simulink model "Smart_Grid_2"  (R2024b)
settings: Solver=FixedStepAuto  StartTime=0.0  StopTime=0.5  FixedStep=1e-5  RelTol=1e-3
undefined symbols (not defined in the file): Ion, Lithium
libraries: spsSeriesRLCBranchLib x76, spsRMSLib x65, spsIGBTDiodeLib x41, eeGeneralControl x36, slpidlib x34, spsThreePhaseVIMeasurementLib x32, spsVoltageMeasurementLib x18, simulink x16, spsCurrentMeasurementLib x15, spsThreePhaseBreakerLib x12, spsAlphaBetaZerotodq0Lib x12, spsPower3phPhasorLib x10
(part 1 of 8)
settings Model: Creator=siva kumar  LastModifiedBy=siva kumar
settings RTWCC: GPUComputeCapability=3.5

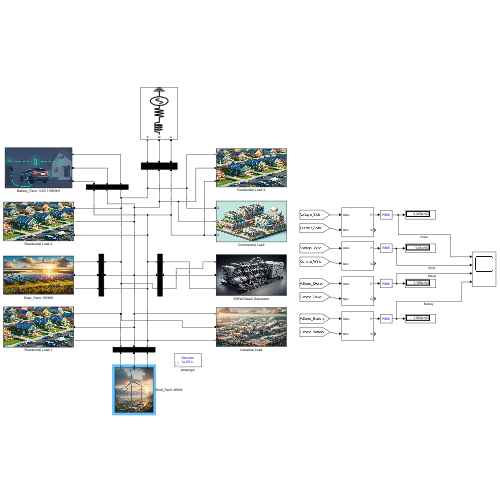
[thumbnail: Simulink's stored preview of the top-level diagram]
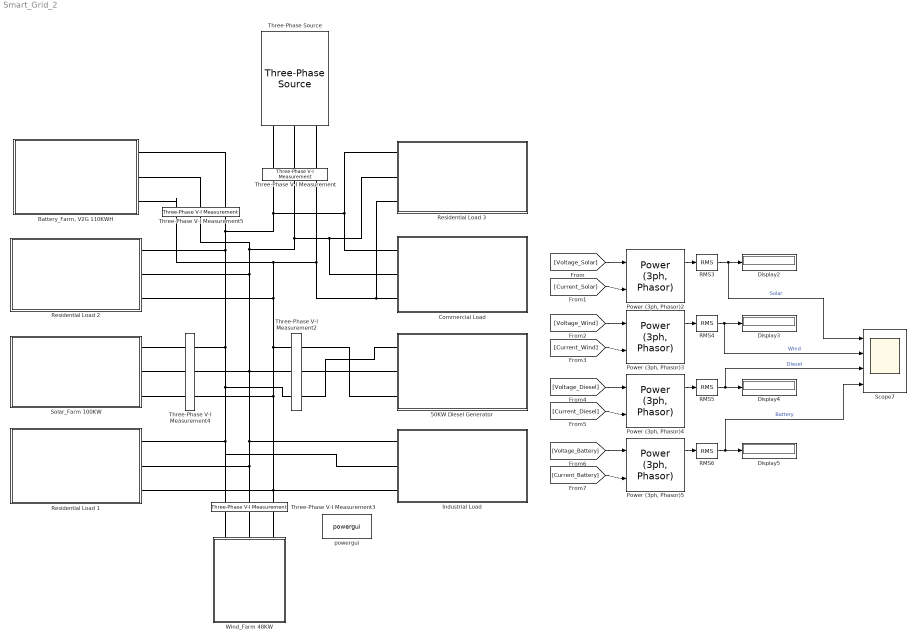
== system Smart_Grid_2 ==
  50KW Diesel Generator : Subsystem
      mask Display: image('Diesel_Image.jpg');
  "Battery_Farm, V2G 110KWH" : Subsystem
      mask Display: image('v2g.png');
  Commercial Load : Subsystem
      mask Display: image('Commercial_Image.jpg');
  Display{2..5} (4 alike) : Display
  Industrial Load : Subsystem
      mask Display: image('Industrial_Image.jpg');
  Power (3ph, Phasor){2..5} (4 alike) : spsPower3phPhasorLib/Power (3ph, Phasor)
      settings: LibrarySourceBlock=|
      | sps_lib/Sensors and Measurements/Power
      | (3ph, Phasor)
  RMS{3..6} (4 alike) : spsRMSLib/RMS  TrueRMS=on  Freq=50  RMSInit=0  Ts=0
  Residential Load 1 : Subsystem
      mask Display: image('Residential_Image.jpg');
  Residential Load 2 : Subsystem
      mask Display: image('Residential_Image.jpg');
  Residential Load 3 : Subsystem
      mask Display: image('Residential_Image.jpg');
  Scope7 : Scope  NumInputPorts=4
  Solar_Farm 100KW : Subsystem
      mask Display: image('Solar_Image.jpg');
  Three-Phase V-I Measurement : spsThreePhaseVIMeasurementLib/Three-Phase V-I Measurement  VoltageMeasurement=phase-to-ground  SetLabelV=on  LabelV=Grid_Voltage  Vpu=off  VpuLL=off  CurrentMeasurement=yes  SetLabelI=on  LabelI=Grid_Current  Ipu=off  Pbase=100e6  Vbase=500e3  OutputType=Complex  PhasorSimulation=off  PSBequivalent=0
  Three-Phase V-I Measurement2 : spsThreePhaseVIMeasurementLib/Three-Phase V-I Measurement  VoltageMeasurement=phase-to-ground  SetLabelV=on  LabelV=Voltage_Diesel  Vpu=off  VpuLL=off  CurrentMeasurement=yes  SetLabelI=on  LabelI=Current_Diesel  Ipu=off  Pbase=100e6  Vbase=500e3  OutputType=Complex  PhasorSimulation=off  PSBequivalent=0
  Three-Phase V-I Measurement3 : spsThreePhaseVIMeasurementLib/Three-Phase V-I Measurement  VoltageMeasurement=phase-to-ground  SetLabelV=on  LabelV=Voltage_Wind  Vpu=off  VpuLL=off  CurrentMeasurement=yes  SetLabelI=on  LabelI=Current_Wind  Ipu=off  Pbase=100e6  Vbase=500e3  OutputType=Complex  PhasorSimulation=off  PSBequivalent=0
  Three-Phase V-I Measurement4 : spsThreePhaseVIMeasurementLib/Three-Phase V-I Measurement  VoltageMeasurement=phase-to-ground  SetLabelV=on  LabelV=Voltage_Solar  Vpu=off  VpuLL=off  CurrentMeasurement=yes  SetLabelI=on  LabelI=Current_Solar  Ipu=off  Pbase=100e6  Vbase=500e3  OutputType=Complex  PhasorSimulation=off  PSBequivalent=0
  Three-Phase V-I Measurement5 : spsThreePhaseVIMeasurementLib/Three-Phase V-I Measurement  VoltageMeasurement=phase-to-ground  SetLabelV=on  LabelV=Voltage_Battery  Vpu=off  VpuLL=off  CurrentMeasurement=yes  SetLabelI=on  LabelI=Current_Battery  Ipu=off  Pbase=100e6  Vbase=500e3  OutputType=Complex  PhasorSimulation=off  PSBequivalent=0
  Three-Phase Source : spsThreePhaseSourceLib/Three-Phase Source  InternalConnection=Yg  VoltagePhases=off  Voltage=25e3  PhaseAngle=0  Voltage_phases=[25e3 25e3 25e3]/sqrt(3)  PhaseAngles_phases=[0 -120 +120]  Frequency=50  NonIdealSource=on  SpecifyImpedance=off  Resistance=0.8929  Inductance=16.58e-3  ShortCircuitLevel=100e6  BaseVoltage=25e3  XRratio=7  BusType=swing  Pref=10e3  Qref=0  Prefabc=[10e3, 10e3, 10e3]  Qrefabc=[0, 0, 0]  Qmin=-inf  Qmax=inf
  Wind_Farm 48KW : Subsystem
      mask Display: image('Wind_Image.jpg');
  powergui : sps_lib/powergui  Priority=1  SimulationMode=Discrete  SampleTime=1e-5  frequency=60  Iterations=50  frequencyindice=0  Pbase=100e6  ErrMax=1e-4  UnitsV=kV  UnitsW=MW  buscounter=0  FunctionMessages=off  echomessages=off  EnableUseOfTLC=off  CurrentSourceSwitches=off  DisableSnubberDevices=off  DisableRonSwitches=off  DisableVfSwitches=off  DisplayEquations=off  AutomaticDiscreteSolvers=off  SolverType=Tustin/Backward Euler (TBE)  Interpol=off  ExternalGateDelay=off  methode=off  Ts=100  x0status=blocks  SPID=on  SwTol=0  HookPort=off  NonlinearTolerance=1e-4  nMaxIteration=100  ContinueOnMaxIteration=off  RestoreLinks=warning  ResistiveCurrentMeasurement=off  Frange=[0:2:500]  Ylog=off  Xlog=on  ShowGrid=off  save=off  variable=ZData  structure=0  ZoomFFT=off  StartTime=0.0  cycles=1  DisplayStyle=1  fundamental=60  FreqAxis=off  MaxFrequency=1000  frequencyindicesteady=1  RmsSteady=1  display=off
  wires:
  RMS3/1 -> Scope7/1, Display2/1  "Solar"
  "Power (3ph, Phasor)2"/1 -> RMS3/1
  [Voltage_Solar] -> "Power (3ph, Phasor)2"/1
  [Current_Solar] -> "Power (3ph, Phasor)2"/2
  [Current_Wind] -> "Power (3ph, Phasor)3"/2
  [Voltage_Wind] -> "Power (3ph, Phasor)3"/1
  "Power (3ph, Phasor)3"/1 -> RMS4/1
  RMS4/1 -> Scope7/2, Display3/1  "Wind"
  RMS5/1 -> Scope7/3, Display4/1  "Diesel"
  "Power (3ph, Phasor)4"/1 -> RMS5/1
  [Voltage_Diesel] -> "Power (3ph, Phasor)4"/1
  [Current_Diesel] -> "Power (3ph, Phasor)4"/2
  [Current_Battery] -> "Power (3ph, Phasor)5"/2
  [Voltage_Battery] -> "Power (3ph, Phasor)5"/1
  "Power (3ph, Phasor)5"/1 -> RMS6/1
  RMS6/1 -> Scope7/4, Display5/1  "Battery"
  connections:
  Three-Phase V-I Measurement3/RConn1 -- Residential Load 2/LConn1 -- Residential Load 3/LConn1 -- Commercial Load/LConn1 -- Three-Phase V-I Measurement/RConn1 -- Three-Phase V-I Measurement5/RConn1 -- Three-Phase V-I Measurement4/RConn1 -- Three-Phase V-I Measurement2/RConn1 -- Industrial Load/LConn2 -- Residential Load 1/LConn1
  Three-Phase V-I Measurement2/RConn3 -- Residential Load 2/LConn3 -- Three-Phase V-I Measurement5/RConn3 -- Residential Load 3/LConn3 -- Commercial Load/LConn3 -- Three-Phase V-I Measurement/RConn3 -- Industrial Load/LConn3 -- Three-Phase V-I Measurement3/RConn3 -- Residential Load 1/LConn3 -- Three-Phase V-I Measurement4/RConn3
  Three-Phase V-I Measurement2/RConn2 -- Residential Load 2/LConn2 -- Three-Phase V-I Measurement5/RConn2 -- Residential Load 3/LConn2 -- Commercial Load/LConn2 -- Three-Phase V-I Measurement/RConn2 -- Three-Phase V-I Measurement3/RConn2 -- Residential Load 1/LConn2 -- Industrial Load/LConn1 -- Three-Phase V-I Measurement4/RConn2
  Three-Phase Source/RConn1 -- Three-Phase V-I Measurement/LConn1
  Three-Phase Source/RConn2 -- Three-Phase V-I Measurement/LConn2
  Three-Phase Source/RConn3 -- Three-Phase V-I Measurement/LConn3
  Wind_Farm 48KW/RConn2 -- Three-Phase V-I Measurement3/LConn2
  Wind_Farm 48KW/RConn1 -- Three-Phase V-I Measurement3/LConn1
  Solar_Farm 100KW/RConn1 -- Three-Phase V-I Measurement4/LConn1
  Solar_Farm 100KW/RConn2 -- Three-Phase V-I Measurement4/LConn2
  Solar_Farm 100KW/RConn3 -- Three-Phase V-I Measurement4/LConn3
  Three-Phase V-I Measurement5/LConn1 -- "Battery_Farm, V2G 110KWH"/RConn1
  Three-Phase V-I Measurement5/LConn2 -- "Battery_Farm, V2G 110KWH"/RConn2
  Three-Phase V-I Measurement5/LConn3 -- "Battery_Farm, V2G 110KWH"/RConn3
  Three-Phase V-I Measurement3/LConn3 -- Wind_Farm 48KW/RConn3
  Three-Phase V-I Measurement2/LConn1 -- 50KW Diesel Generator/RConn1
  Three-Phase V-I Measurement2/LConn2 -- 50KW Diesel Generator/RConn2
  Three-Phase V-I Measurement2/LConn3 -- 50KW Diesel Generator/RConn3

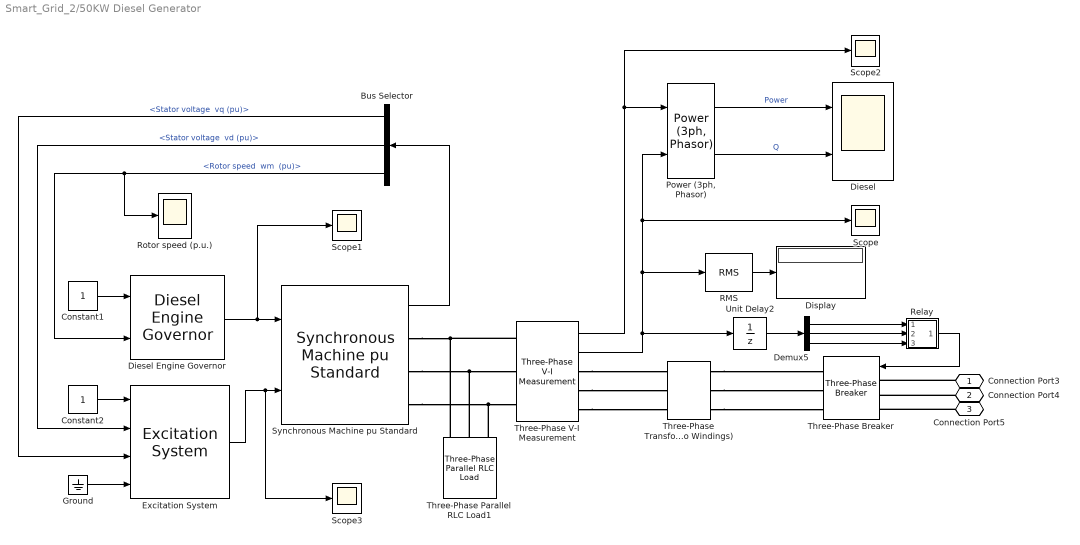
== system Smart_Grid_2/50KW Diesel Generator ==
  Bus Selector : BusSelector  OutputSignals="dq0 components.Stator voltage  vq (pu),dq0 components.Stator voltage  vd (pu),Mechanical.Rotor speed  wm  (pu)"
  Constant1 : Constant
  Constant2 : Constant
  Demux5 : Demux  Outputs=3
  Diesel : Scope  NumInputPorts=2
  Diesel Engine Governor : spsDieselMotorModel/Diesel Engine Governor  K=65  Tr=[0.01 0.02 0.2]  Ta=[0.25 0.009 0.0384]  Tlim=[0.1 1.1]  Td=0.020  Pm0=0.007343
  Display : Display
  Excitation System : spsExcitationSystemLib/Excitation System  tr=20e-3  reg=[ 300, 0.001 ]  exc=[ 1, 0 ]  tgr=[ 0, 0 ]  damp=[ 0.001, 0.1 ]  sat=[ 0, 0 ]  lim=[ -11.5, 11.5, 0 ]  v0=[1 1.0072]
      settings: LibrarySourceBlock=sps_lib/Electrical Machines/Synchronous Machine Control/Excitation System
  Ground : Ground
  "Power (3ph, Phasor)" : spsPower3phPhasorLib/Power (3ph, Phasor)
      settings: LibrarySourceBlock=|
      | sps_lib/Sensors and Measurements/Power
      | (3ph, Phasor)
  RMS : spsRMSLib/RMS  TrueRMS=on  Freq=50  RMSInit=0  Ts=0.001
  Relay : Subsystem
  Rotor speed (p.u.) : Scope
  Scope{,1..3} (4 alike) : Scope
  Synchronous Machine pu Standard : spsSynchronousMachinepuStandardLib/Synchronous Machine pu Standard  PresetModel=No  MechanicalLoad=Mechanical power Pm  ShowDetailedParameters=on  RotorType=Salient-pole  Units=per unit standard parameters  MeasurementBus=off  NominalParameters="[ 150e3  25e3   50]"  Reactances1=[ 1.81, 0.3, 0.23, 1.76, 0.65, 0.25, 0.15 ]  Reactances2="[ 1.305, 0.296, 0.252, 0.474,  0.243,  0.18 ]"  dAxisTimeConstants=Open-circuit  qAxisTimeConstants=Short-circuit  TimeConstants1="[ 4.4849  0.0681  0.1  ]"  TimeConstants2=[ 8.0, 0.03, 1.0, 0.07 ]  TimeConstants3="[  4.49  0.0681  0.0513  ]"  TimeConstants4=[ 8.0, 0.03, 0.3371, 0.0295 ]  TimeConstants5=[ 1.01, 0.053, 0.1 ]  TimeConstants6=[ 1.3201, 0.023, 1.0, 0.07 ]  TimeConstants7=[0.012 0.003 0.003]  TimeConstants8=[ 1.3201, 0.0231, 0.3371, 0.0295 ]  StatorResistance=0.003  Mechanical=[3.7 0 1 ]  PolePairs=20  InitialConditions=[0 -89.802 0.00913935 0.00913935 0.00913935 -36.542 -156.542 83.458 1.00715]  SetSaturation=off  Saturation=[0.6404,0.7127,0.8441,0.9214,0.9956,1.082,1.19,1.316,1.457;0.7,0.7698,0.8872,0.9466,0.9969,1.046,1.1,1.151,1.201]  LoadFlowParameters=[1,0,0,0,0]  TsPowergui=0  TsBlock=-1  IterativeModel=Trapezoidal non iterative  IterativeDiscreteModel=Trapezoidal non iterative  BusType=swing  Pref=0  Qref=0  Qmin=-inf  Qmax=inf  PLF=0  QLF=0
  Three-Phase Parallel RLC Load1 : spsThreePhaseParallelRLCLoadLib/Three-Phase Parallel RLC Load  LConnTagsString=A|B|C  Configuration=Y (floating)  NominalVoltage=(25000*sqrt(3))*1  Vabc=[1e3 1e3 1e3]  Vabcp=[1e3 1e3 1e3]  NominalFrequency=50  UnbalancedPower=off  ActivePower=1e3  InductivePower=0  CapacitivePower=0  Pabc=[10e3 9e3 11e3]  QLabc=[100 90 110]  QCabc=[100 90 110]  Pabcp=[10e3 9e3 11e3]  QLabcp=[100 90 110]  QCabcp=[100 90 110]  Measurements=None  LoadType=constant PQ
  Three-Phase Transformer (Two Windings) : spsThreePhaseTransformerTwoWindingsLib/Three-Phase Transformer (Two Windings)  Winding1Connection=Yg  Winding2Connection=Yg  CoreType=Three single-phase transformers  SetSaturation=off  Hysteresis=off  DataFile='hysteresis'  SetInitialFlux=off  Measurements=None  UNITS=pu  NominalPower=[ 200e3 , 50 ]  Winding1=[ 25e3 , 0.002 , 0.08 ]  Winding2=[ 25e3 , 0.002 , 0.08 ]  Rm=500  Lm=500  L0=0.5  Saturation=[ 0,0 ; 0.0024,1.2 ; 1.0,1.52 ]  InitialFluxes=[ 0.8 , -0.8 , 0.7 ]  BreakLoop=off  DiscreteSolver=Trapezoidal iterative  DataType=off  TransfoNumber=1
  Three-Phase V-I Measurement : spsThreePhaseVIMeasurementLib/Three-Phase V-I Measurement  VoltageMeasurement=phase-to-ground  SetLabelV=off  LabelV=Vabc  Vpu=off  VpuLL=off  CurrentMeasurement=yes  SetLabelI=off  LabelI=Iabc  Ipu=off  Pbase=100e6  Vbase=500e3  OutputType=Complex  PhasorSimulation=off  PSBequivalent=0
  Three-Phase Breaker : spsThreePhaseBreakerLib/Three-Phase Breaker  InitialState=closed  SwitchA=on  SwitchB=on  SwitchC=on  SwitchTimes="[1/60  5/60]"  External=on  BreakerResistance=0.001  SnubberResistance=1e8  SnubberCapacitance=inf  Measurements=Breaker voltages and currents
  Unit Delay2 : UnitDelay  SampleTime=0.001  HasFrameUpgradeWarning=on
  Connection Port3 : PMIOPort  Side=Right
  Connection Port4 : PMIOPort  Port=2  Side=Right
  Connection Port5 : PMIOPort  Port=3  Side=Right
  wires:
  Demux5/3 -> Relay/3(In3)
  Relay/1(Out1) -> Three-Phase Breaker/1
  Bus Selector/1 -> Excitation System/3  "<Stator voltage  vq (pu)>"
  Bus Selector/2 -> Excitation System/2  "<Stator voltage  vd (pu)>"
  Three-Phase V-I Measurement/2 -> Unit Delay2/1, "Power (3ph, Phasor)"/2, Scope/1, RMS/1
  "Power (3ph, Phasor)"/1 -> Diesel/1  "Power"
  Three-Phase V-I Measurement/1 -> Scope2/1, "Power (3ph, Phasor)"/1
  Excitation System/1 -> Scope3/1, Synchronous Machine pu Standard/2
  "Power (3ph, Phasor)"/2 -> Diesel/2  "Q"
  RMS/1 -> Display/1
  Ground/1 -> Excitation System/4
  Bus Selector/3 -> Rotor speed (p.u.)/1, Diesel Engine Governor/2  "<Rotor speed  wm  (pu)>"
  Synchronous Machine pu Standard/1 -> Bus Selector/1
  Constant2/1 -> Excitation System/1
  Demux5/2 -> Relay/2(In2)
  Diesel Engine Governor/1 -> Scope1/1, Synchronous Machine pu Standard/1
  Demux5/1 -> Relay/1(In1)
  Unit Delay2/1 -> Demux5/1
  Constant1/1 -> Diesel Engine Governor/1
  connections:
  Synchronous Machine pu Standard/RConn3 -- Three-Phase Parallel RLC Load1/LConn3 -- Three-Phase V-I Measurement/LConn3
  Synchronous Machine pu Standard/RConn1 -- Three-Phase Parallel RLC Load1/LConn1 -- Three-Phase V-I Measurement/LConn1
  Synchronous Machine pu Standard/RConn2 -- Three-Phase Parallel RLC Load1/LConn2 -- Three-Phase V-I Measurement/LConn2
  Connection Port4/RConn1 -- Three-Phase Breaker/LConn2
  Connection Port3/RConn1 -- Three-Phase Breaker/LConn1
  Connection Port5/RConn1 -- Three-Phase Breaker/LConn3
  Three-Phase V-I Measurement/RConn1 -- Three-Phase Transformer (Two Windings)/LConn1
  Three-Phase V-I Measurement/RConn2 -- Three-Phase Transformer (Two Windings)/LConn2
  Three-Phase V-I Measurement/RConn3 -- Three-Phase Transformer (Two Windings)/LConn3
  Three-Phase Transformer (Two Windings)/RConn1 -- Three-Phase Breaker/RConn1
  Three-Phase Transformer (Two Windings)/RConn2 -- Three-Phase Breaker/RConn2
  Three-Phase Transformer (Two Windings)/RConn3 -- Three-Phase Breaker/RConn3

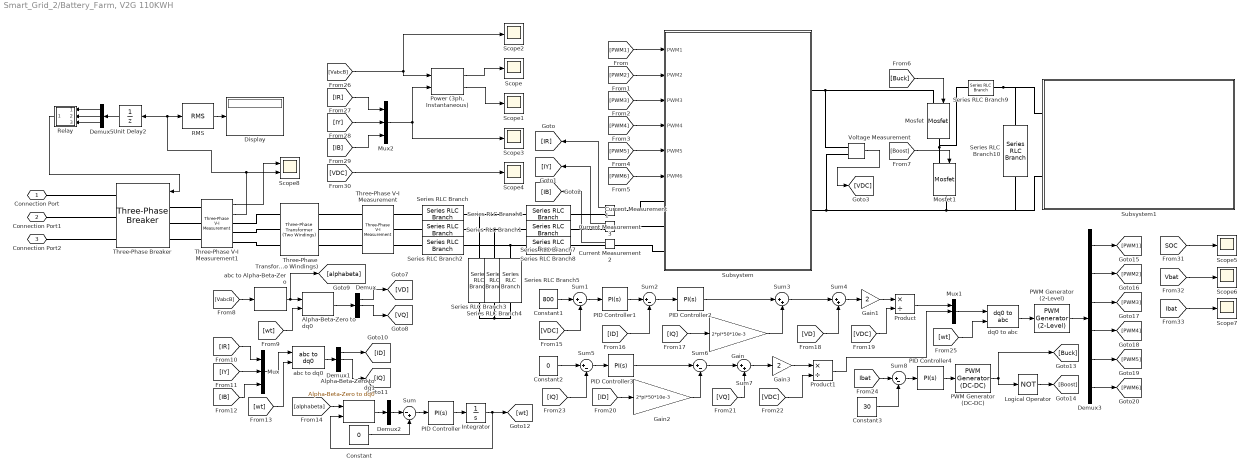
== system Smart_Grid_2/Battery_Farm, V2G 110KWH ==
  Alpha-Beta-Zero to dq0 : spsAlphaBetaZerotodq0Lib/Alpha-Beta-Zero to dq0  Alignment=90 degrees behind phase A axis
  Alpha-Beta-Zero to dq1 : spsAlphaBetaZerotodq0Lib/Alpha-Beta-Zero to dq0  Alignment=90 degrees behind phase A axis
  Constant : Constant  Value=0
  Constant1 : Constant  Value=800
  Constant2 : Constant  Value=0
  Constant3 : Constant  Value=30
  Current Measurement1 : spsCurrentMeasurementLib/Current Measurement  PhasorSimulation=off  OutputType=Complex  PSBequivalent=0
  Current Measurement2 : spsCurrentMeasurementLib/Current Measurement  PhasorSimulation=off  OutputType=Complex  PSBequivalent=0
  Current Measurement3 : spsCurrentMeasurementLib/Current Measurement  PhasorSimulation=off  OutputType=Complex  PSBequivalent=0
  Demux{,1..2,5} (4 alike) : Demux  Outputs=3
  Demux3 : Demux  Outputs=6
  Display : Display
  Gain : Gain  Gain=2*pi*50*10e-3
  Gain1 : Gain  Gain=2
  Gain2 : Gain  Gain=2*pi*50*10e-3
  Gain3 : Gain  Gain=2
  Integrator : Integrator
  Logical Operator : Logic  Operator=NOT  AllPortsSameDT=off  OutDataTypeStr=boolean
  Mosfet : spsMosfetLib/Mosfet  Ron=0.1  Lon=0  Rd=0.01  Vfd=0  IC=0  Rs=1e5  Cs=inf  Measurements=off
  Mosfet1 : spsMosfetLib/Mosfet  Ron=0.1  Lon=0  Rd=0.01  Vfd=0  IC=0  Rs=1e5  Cs=inf  Measurements=off
  Mux : Mux  Inputs=3
  Mux1 : Mux  Inputs=3
  Mux2 : Mux  Inputs=3
  PID Controller : slpidlib/PID Controller  Controller=PI  Form=Parallel  TimeDomain=Continuous-time  UseExternalTs=off  SampleTime=-1  IntegratorMethod=Forward Euler  FilterMethod=Forward Euler  ControllerParametersSource=internal  P=10  I=50000  UseKiTs=off  D=0  UseExternalDerivativeSource=off  N=100  UseFilter=on  TunerSelectOption=Transfer Function Based (PID Tuner App)  InitialConditionSource=internal  InitialConditionForIntegrator=0  InitialConditionForFilter=0  DifferentiatorICPrevScaledInput=0  ExternalReset=none  TrackingMode=off  Kt=1  LimitOutput=off  SatLimitsSource=internal  UpperSaturationLimit=inf  LowerSaturationLimit=-inf  LinearizeAsGain=on  AntiWindupMode=none  Kb=1  LimitIntegrator=off  UpperIntegratorSaturationLimit=inf  LowerIntegratorSaturationLimit=-inf  POutMin=[]  POutMax=[]  IOutMin=[]  IOutMax=[]  DOutMin=[]  DOutMax=[]  NOutMin=[]  NOutMax=[]  SumOutMin=[]  SumOutMax=[]  SaturationOutMin=[]  SaturationOutMax=[]  PParamMin=[]  PParamMax=[]  IParamMin=[]  IParamMax=[]  DParamMin=[]  DParamMax=[]  NParamMin=[]  NParamMax=[]  KbParamMin=[]  KbParamMax=[]  KtParamMin=[]  KtParamMax=[]  KbOutMin=[]  KbOutMax=[]  KtOutMin=[]  KtOutMax=[]  IntegratorOutMin=[]  IntegratorOutMax=[]  FilterOutMin=[]  FilterOutMax=[]  SumI1OutMin=[]  SumI1OutMax=[]  SumI2OutMin=[]  SumI2OutMax=[]  SumI3OutMin=[]  SumI3OutMax=[]  SumI4OutMin=[]  SumI4OutMax=[]  SumDOutMin=[]  SumDOutMax=[]  DifferentiatorOutMin=[]  DifferentiatorOutMax=[]  FilterDiffOutCoefMin=[]  FilterDiffOutCoefMax=[]  ReciprocalOutMin=[]  ReciprocalOutMax=[]  SumDenOutMin=[]  SumDenOutMax=[]  SumNumOutMin=[]  SumNumOutMax=[]  DivideOutMin=[]  DivideOutMax=[]  UdiffTsProdOutMin=[]  UdiffTsProdOutMax=[]  NTsProdOutMin=[]  NTsProdOutMax=[]  UintegralTsProdOutMin=[]  UintegralTsProdOutMax=[]  UngainTsProdOutMin=[]  UngainTsProdOutMax=[]  ClampingZeroOutDataTypeStr=Inherit: Inherit via back propagation  ClampingZeroOutMin=[]  ClampingZeroOutMax=[]  FilterDenConstantOutDataTypeStr=Inherit: Inherit via back propagation  FilterDenConstantOutMin=[]  FilterDenConstantOutMax=[]  PCopyOutDataTypeStr=Inherit: Inherit via back propagation  PCopyOutMin=[]  PCopyOutMax=[]  NCopyOutDataTypeStr=Inherit: Inherit via back propagation  NCopyOutMin=[]  NCopyOutMax=[]  IntegratorContinuousStateAttributes=''  IntegratorStateMustResolveToSignalObject=off  IntegratorRTWStateStorageClass=Auto  FilterContinuousStateAttributes=''  FilterStateMustResolveToSignalObject=off  FilterRTWStateStorageClass=Auto  ParallelPVariant=InternalParameters  IdealPVariant=Disabled  IVariant=InternalParameters  DVariant=Disabled  IntegratorVariant=Continuous  SatVariant=Disabled  AWVariant=Passthrough  PCopyVariant=Disabled  TRVariant=Disabled  FdbkBlocksVariant=Forward  IdealPFdbkVariant=Disabled  SatFdbkVariant=Disabled  DerivativeFilterVariant=Disabled  NVariant=Disabled  NCopyVariant=Disabled_SignalSpec  FilterICVariant=Disabled  IntegratorICVariant=InternalICs  ExternalResetVariant=Disabled  TRSumVariant=Passthrough  SumFdbkVariant=Disabled  SumVariant=Sum_PI  TsampFilterVariant=InternalTs  TsampNgainVariant=Passthrough  TsampIntegralVariant=Disabled_SignalSpec  ExternalSaturationOutDataTypeStr=Inherit: Same as second input  DerivativeSourceVariant=Disabled  PreIntVariant=InternalPreInt
  PID Controller1 : slpidlib/PID Controller  Controller=PI  Form=Parallel  TimeDomain=Continuous-time  UseExternalTs=off  SampleTime=-1  IntegratorMethod=Forward Euler  FilterMethod=Forward Euler  ControllerParametersSource=internal  P=0.5  I=5  UseKiTs=off  D=0  UseExternalDerivativeSource=off  N=100  UseFilter=on  TunerSelectOption=Transfer Function Based (PID Tuner App)  InitialConditionSource=internal  InitialConditionForIntegrator=0  InitialConditionForFilter=0  DifferentiatorICPrevScaledInput=0  ExternalReset=none  TrackingMode=off  Kt=1  LimitOutput=off  SatLimitsSource=internal  UpperSaturationLimit=inf  LowerSaturationLimit=-inf  LinearizeAsGain=on  AntiWindupMode=none  Kb=1  LimitIntegrator=off  UpperIntegratorSaturationLimit=inf  LowerIntegratorSaturationLimit=-inf  POutMin=[]  POutMax=[]  IOutMin=[]  IOutMax=[]  DOutMin=[]  DOutMax=[]  NOutMin=[]  NOutMax=[]  SumOutMin=[]  SumOutMax=[]  SaturationOutMin=[]  SaturationOutMax=[]  PParamMin=[]  PParamMax=[]  IParamMin=[]  IParamMax=[]  DParamMin=[]  DParamMax=[]  NParamMin=[]  NParamMax=[]  KbParamMin=[]  KbParamMax=[]  KtParamMin=[]  KtParamMax=[]  KbOutMin=[]  KbOutMax=[]  KtOutMin=[]  KtOutMax=[]  IntegratorOutMin=[]  IntegratorOutMax=[]  FilterOutMin=[]  FilterOutMax=[]  SumI1OutMin=[]  SumI1OutMax=[]  SumI2OutMin=[]  SumI2OutMax=[]  SumI3OutMin=[]  SumI3OutMax=[]  SumI4OutMin=[]  SumI4OutMax=[]  SumDOutMin=[]  SumDOutMax=[]  DifferentiatorOutMin=[]  DifferentiatorOutMax=[]  FilterDiffOutCoefMin=[]  FilterDiffOutCoefMax=[]  ReciprocalOutMin=[]  ReciprocalOutMax=[]  SumDenOutMin=[]  SumDenOutMax=[]  SumNumOutMin=[]  SumNumOutMax=[]  DivideOutMin=[]  DivideOutMax=[]  UdiffTsProdOutMin=[]  UdiffTsProdOutMax=[]  NTsProdOutMin=[]  NTsProdOutMax=[]  UintegralTsProdOutMin=[]  UintegralTsProdOutMax=[]  UngainTsProdOutMin=[]  UngainTsProdOutMax=[]  ClampingZeroOutDataTypeStr=Inherit: Inherit via back propagation  ClampingZeroOutMin=[]  ClampingZeroOutMax=[]  FilterDenConstantOutDataTypeStr=Inherit: Inherit via back propagation  FilterDenConstantOutMin=[]  FilterDenConstantOutMax=[]  PCopyOutDataTypeStr=Inherit: Inherit via back propagation  PCopyOutMin=[]  PCopyOutMax=[]  NCopyOutDataTypeStr=Inherit: Inherit via back propagation  NCopyOutMin=[]  NCopyOutMax=[]  IntegratorContinuousStateAttributes=''  IntegratorStateMustResolveToSignalObject=off  IntegratorRTWStateStorageClass=Auto  FilterContinuousStateAttributes=''  FilterStateMustResolveToSignalObject=off  FilterRTWStateStorageClass=Auto  ParallelPVariant=InternalParameters  IdealPVariant=Disabled  IVariant=InternalParameters  DVariant=Disabled  IntegratorVariant=Continuous  SatVariant=Disabled  AWVariant=Passthrough  PCopyVariant=Disabled  TRVariant=Disabled  FdbkBlocksVariant=Forward  IdealPFdbkVariant=Disabled  SatFdbkVariant=Disabled  DerivativeFilterVariant=Disabled  NVariant=Disabled  NCopyVariant=Disabled_SignalSpec  FilterICVariant=Disabled  IntegratorICVariant=InternalICs  ExternalResetVariant=Disabled  TRSumVariant=Passthrough  SumFdbkVariant=Disabled  SumVariant=Sum_PI  TsampFilterVariant=InternalTs  TsampNgainVariant=Passthrough  TsampIntegralVariant=Disabled_SignalSpec  ExternalSaturationOutDataTypeStr=Inherit: Same as second input  DerivativeSourceVariant=Disabled  PreIntVariant=InternalPreInt
  PID Controller2 : slpidlib/PID Controller  Controller=PI  Form=Parallel  TimeDomain=Continuous-time  UseExternalTs=off  SampleTime=-1  IntegratorMethod=Forward Euler  FilterMethod=Forward Euler  ControllerParametersSource=internal  P=25  I=500  UseKiTs=off  D=0  UseExternalDerivativeSource=off  N=100  UseFilter=on  TunerSelectOption=Transfer Function Based (PID Tuner App)  InitialConditionSource=internal  InitialConditionForIntegrator=0  InitialConditionForFilter=0  DifferentiatorICPrevScaledInput=0  ExternalReset=none  TrackingMode=off  Kt=1  LimitOutput=off  SatLimitsSource=internal  UpperSaturationLimit=inf  LowerSaturationLimit=-inf  LinearizeAsGain=on  AntiWindupMode=none  Kb=1  LimitIntegrator=off  UpperIntegratorSaturationLimit=inf  LowerIntegratorSaturationLimit=-inf  POutMin=[]  POutMax=[]  IOutMin=[]  IOutMax=[]  DOutMin=[]  DOutMax=[]  NOutMin=[]  NOutMax=[]  SumOutMin=[]  SumOutMax=[]  SaturationOutMin=[]  SaturationOutMax=[]  PParamMin=[]  PParamMax=[]  IParamMin=[]  IParamMax=[]  DParamMin=[]  DParamMax=[]  NParamMin=[]  NParamMax=[]  KbParamMin=[]  KbParamMax=[]  KtParamMin=[]  KtParamMax=[]  KbOutMin=[]  KbOutMax=[]  KtOutMin=[]  KtOutMax=[]  IntegratorOutMin=[]  IntegratorOutMax=[]  FilterOutMin=[]  FilterOutMax=[]  SumI1OutMin=[]  SumI1OutMax=[]  SumI2OutMin=[]  SumI2OutMax=[]  SumI3OutMin=[]  SumI3OutMax=[]  SumI4OutMin=[]  SumI4OutMax=[]  SumDOutMin=[]  SumDOutMax=[]  DifferentiatorOutMin=[]  DifferentiatorOutMax=[]  FilterDiffOutCoefMin=[]  FilterDiffOutCoefMax=[]  ReciprocalOutMin=[]  ReciprocalOutMax=[]  SumDenOutMin=[]  SumDenOutMax=[]  SumNumOutMin=[]  SumNumOutMax=[]  DivideOutMin=[]  DivideOutMax=[]  UdiffTsProdOutMin=[]  UdiffTsProdOutMax=[]  NTsProdOutMin=[]  NTsProdOutMax=[]  UintegralTsProdOutMin=[]  UintegralTsProdOutMax=[]  UngainTsProdOutMin=[]  UngainTsProdOutMax=[]  ClampingZeroOutDataTypeStr=Inherit: Inherit via back propagation  ClampingZeroOutMin=[]  ClampingZeroOutMax=[]  FilterDenConstantOutDataTypeStr=Inherit: Inherit via back propagation  FilterDenConstantOutMin=[]  FilterDenConstantOutMax=[]  PCopyOutDataTypeStr=Inherit: Inherit via back propagation  PCopyOutMin=[]  PCopyOutMax=[]  NCopyOutDataTypeStr=Inherit: Inherit via back propagation  NCopyOutMin=[]  NCopyOutMax=[]  IntegratorContinuousStateAttributes=''  IntegratorStateMustResolveToSignalObject=off  IntegratorRTWStateStorageClass=Auto  FilterContinuousStateAttributes=''  FilterStateMustResolveToSignalObject=off  FilterRTWStateStorageClass=Auto  ParallelPVariant=InternalParameters  IdealPVariant=Disabled  IVariant=InternalParameters  DVariant=Disabled  IntegratorVariant=Continuous  SatVariant=Disabled  AWVariant=Passthrough  PCopyVariant=Disabled  TRVariant=Disabled  FdbkBlocksVariant=Forward  IdealPFdbkVariant=Disabled  SatFdbkVariant=Disabled  DerivativeFilterVariant=Disabled  NVariant=Disabled  NCopyVariant=Disabled_SignalSpec  FilterICVariant=Disabled  IntegratorICVariant=InternalICs  ExternalResetVariant=Disabled  TRSumVariant=Passthrough  SumFdbkVariant=Disabled  SumVariant=Sum_PI  TsampFilterVariant=InternalTs  TsampNgainVariant=Passthrough  TsampIntegralVariant=Disabled_SignalSpec  ExternalSaturationOutDataTypeStr=Inherit: Same as second input  DerivativeSourceVariant=Disabled  PreIntVariant=InternalPreInt
  PID Controller3 : slpidlib/PID Controller  Controller=PI  Form=Parallel  TimeDomain=Continuous-time  UseExternalTs=off  SampleTime=-1  IntegratorMethod=Forward Euler  FilterMethod=Forward Euler  ControllerParametersSource=internal  P=25  I=500  UseKiTs=off  D=0  UseExternalDerivativeSource=off  N=100  UseFilter=on  TunerSelectOption=Transfer Function Based (PID Tuner App)  InitialConditionSource=internal  InitialConditionForIntegrator=0  InitialConditionForFilter=0  DifferentiatorICPrevScaledInput=0  ExternalReset=none  TrackingMode=off  Kt=1  LimitOutput=off  SatLimitsSource=internal  UpperSaturationLimit=inf  LowerSaturationLimit=-inf  LinearizeAsGain=on  AntiWindupMode=none  Kb=1  LimitIntegrator=off  UpperIntegratorSaturationLimit=inf  LowerIntegratorSaturationLimit=-inf  POutMin=[]  POutMax=[]  IOutMin=[]  IOutMax=[]  DOutMin=[]  DOutMax=[]  NOutMin=[]  NOutMax=[]  SumOutMin=[]  SumOutMax=[]  SaturationOutMin=[]  SaturationOutMax=[]  PParamMin=[]  PParamMax=[]  IParamMin=[]  IParamMax=[]  DParamMin=[]  DParamMax=[]  NParamMin=[]  NParamMax=[]  KbParamMin=[]  KbParamMax=[]  KtParamMin=[]  KtParamMax=[]  KbOutMin=[]  KbOutMax=[]  KtOutMin=[]  KtOutMax=[]  IntegratorOutMin=[]  IntegratorOutMax=[]  FilterOutMin=[]  FilterOutMax=[]  SumI1OutMin=[]  SumI1OutMax=[]  SumI2OutMin=[]  SumI2OutMax=[]  SumI3OutMin=[]  SumI3OutMax=[]  SumI4OutMin=[]  SumI4OutMax=[]  SumDOutMin=[]  SumDOutMax=[]  DifferentiatorOutMin=[]  DifferentiatorOutMax=[]  FilterDiffOutCoefMin=[]  FilterDiffOutCoefMax=[]  ReciprocalOutMin=[]  ReciprocalOutMax=[]  SumDenOutMin=[]  SumDenOutMax=[]  SumNumOutMin=[]  SumNumOutMax=[]  DivideOutMin=[]  DivideOutMax=[]  UdiffTsProdOutMin=[]  UdiffTsProdOutMax=[]  NTsProdOutMin=[]  NTsProdOutMax=[]  UintegralTsProdOutMin=[]  UintegralTsProdOutMax=[]  UngainTsProdOutMin=[]  UngainTsProdOutMax=[]  ClampingZeroOutDataTypeStr=Inherit: Inherit via back propagation  ClampingZeroOutMin=[]  ClampingZeroOutMax=[]  FilterDenConstantOutDataTypeStr=Inherit: Inherit via back propagation  FilterDenConstantOutMin=[]  FilterDenConstantOutMax=[]  PCopyOutDataTypeStr=Inherit: Inherit via back propagation  PCopyOutMin=[]  PCopyOutMax=[]  NCopyOutDataTypeStr=Inherit: Inherit via back propagation  NCopyOutMin=[]  NCopyOutMax=[]  IntegratorContinuousStateAttributes=''  IntegratorStateMustResolveToSignalObject=off  IntegratorRTWStateStorageClass=Auto  FilterContinuousStateAttributes=''  FilterStateMustResolveToSignalObject=off  FilterRTWStateStorageClass=Auto  ParallelPVariant=InternalParameters  IdealPVariant=Disabled  IVariant=InternalParameters  DVariant=Disabled  IntegratorVariant=Continuous  SatVariant=Disabled  AWVariant=Passthrough  PCopyVariant=Disabled  TRVariant=Disabled  FdbkBlocksVariant=Forward  IdealPFdbkVariant=Disabled  SatFdbkVariant=Disabled  DerivativeFilterVariant=Disabled  NVariant=Disabled  NCopyVariant=Disabled_SignalSpec  FilterICVariant=Disabled  IntegratorICVariant=InternalICs  ExternalResetVariant=Disabled  TRSumVariant=Passthrough  SumFdbkVariant=Disabled  SumVariant=Sum_PI  TsampFilterVariant=InternalTs  TsampNgainVariant=Passthrough  TsampIntegralVariant=Disabled_SignalSpec  ExternalSaturationOutDataTypeStr=Inherit: Same as second input  DerivativeSourceVariant=Disabled  PreIntVariant=InternalPreInt
  PID Controller4 : slpidlib/PID Controller  Controller=PI  Form=Parallel  TimeDomain=Continuous-time  UseExternalTs=off  SampleTime=-1  IntegratorMethod=Forward Euler  FilterMethod=Forward Euler  ControllerParametersSource=internal  P=0.005  I=10  UseKiTs=off  D=0  UseExternalDerivativeSource=off  N=100  UseFilter=on  TunerSelectOption=Transfer Function Based (PID Tuner App)  InitialConditionSource=internal  InitialConditionForIntegrator=0  InitialConditionForFilter=0  DifferentiatorICPrevScaledInput=0  ExternalReset=none  TrackingMode=off  Kt=1  LimitOutput=on  SatLimitsSource=internal  UpperSaturationLimit=0.95  LowerSaturationLimit=0  LinearizeAsGain=on  AntiWindupMode=none  Kb=1  LimitIntegrator=off  UpperIntegratorSaturationLimit=inf  LowerIntegratorSaturationLimit=-inf  POutMin=[]  POutMax=[]  IOutMin=[]  IOutMax=[]  DOutMin=[]  DOutMax=[]  NOutMin=[]  NOutMax=[]  SumOutMin=[]  SumOutMax=[]  SaturationOutMin=[]  SaturationOutMax=[]  PParamMin=[]  PParamMax=[]  IParamMin=[]  IParamMax=[]  DParamMin=[]  DParamMax=[]  NParamMin=[]  NParamMax=[]  KbParamMin=[]  KbParamMax=[]  KtParamMin=[]  KtParamMax=[]  KbOutMin=[]  KbOutMax=[]  KtOutMin=[]  KtOutMax=[]  IntegratorOutMin=[]  IntegratorOutMax=[]  FilterOutMin=[]  FilterOutMax=[]  SumI1OutMin=[]  SumI1OutMax=[]  SumI2OutMin=[]  SumI2OutMax=[]  SumI3OutMin=[]  SumI3OutMax=[]  SumI4OutMin=[]  SumI4OutMax=[]  SumDOutMin=[]  SumDOutMax=[]  DifferentiatorOutMin=[]  DifferentiatorOutMax=[]  FilterDiffOutCoefMin=[]  FilterDiffOutCoefMax=[]  ReciprocalOutMin=[]  ReciprocalOutMax=[]  SumDenOutMin=[]  SumDenOutMax=[]  SumNumOutMin=[]  SumNumOutMax=[]  DivideOutMin=[]  DivideOutMax=[]  UdiffTsProdOutMin=[]  UdiffTsProdOutMax=[]  NTsProdOutMin=[]  NTsProdOutMax=[]  UintegralTsProdOutMin=[]  UintegralTsProdOutMax=[]  UngainTsProdOutMin=[]  UngainTsProdOutMax=[]  ClampingZeroOutDataTypeStr=Inherit: Inherit via back propagation  ClampingZeroOutMin=[]  ClampingZeroOutMax=[]  FilterDenConstantOutDataTypeStr=Inherit: Inherit via back propagation  FilterDenConstantOutMin=[]  FilterDenConstantOutMax=[]  PCopyOutDataTypeStr=Inherit: Inherit via back propagation  PCopyOutMin=[]  PCopyOutMax=[]  NCopyOutDataTypeStr=Inherit: Inherit via back propagation  NCopyOutMin=[]  NCopyOutMax=[]  IntegratorContinuousStateAttributes=''  IntegratorStateMustResolveToSignalObject=off  IntegratorRTWStateStorageClass=Auto  FilterContinuousStateAttributes=''  FilterStateMustResolveToSignalObject=off  FilterRTWStateStorageClass=Auto  ParallelPVariant=InternalParameters  IdealPVariant=Disabled  IVariant=InternalParameters  DVariant=Disabled  IntegratorVariant=Continuous  SatVariant=Enabled  AWVariant=Passthrough  PCopyVariant=Disabled  TRVariant=Disabled  FdbkBlocksVariant=Forward  IdealPFdbkVariant=Disabled  SatFdbkVariant=Disabled  DerivativeFilterVariant=Disabled  NVariant=Disabled  NCopyVariant=Disabled_SignalSpec  FilterICVariant=Disabled  IntegratorICVariant=InternalICs  ExternalResetVariant=Disabled  TRSumVariant=Passthrough  SumFdbkVariant=Disabled  SumVariant=Sum_PI  TsampFilterVariant=InternalTs  TsampNgainVariant=Passthrough  TsampIntegralVariant=Disabled_SignalSpec  ExternalSaturationOutDataTypeStr=Inherit: Same as second input  DerivativeSourceVariant=Disabled  PreIntVariant=InternalPreInt
  PWM Generator (2-Level) : spsPWMGenerator2LevelLib/PWM Generator (2-Level)  ModulatorType=Three-phase bridge (6 pulses)  ModulatorMode=Unsynchronized  Fc=10000  Pc=90  nF=27  MinMax="[ -1  1 ]"  SamplingTechnique=Natural  ModulatingSignals=off  m=0.8  Freq=60  Phase=0  Ts=1e-5  ShowCarrierOutport=off
  PWM Generator (DC-DC) : spsPWMGeneratorDCDCLib/PWM Generator (DC-DC)  Fsw=10000  Ts=1e-5
  "Power (3ph, Instantaneous)" : spsPower3phInstantaneousLib/Power (3ph, Instantaneous)
  Product : Product  Inputs=*/
  Product1 : Product  Inputs=*/
  RMS : spsRMSLib/RMS  TrueRMS=on  Freq=50  RMSInit=0  Ts=0.001
  Relay : Subsystem
  Scope{,1..7} (8 alike) : Scope
  Scope8 : Scope  NumInputPorts=2
  Series RLC Branch{,1..2,6..8} (6 alike) : spsSeriesRLCBranchLib/Series RLC Branch  LConnTagsString=__new0  RConnTagsString=__new0  BranchType=L  Resistance=1  Inductance=5e-3  SetiL0=off  InitialCurrent=0  Capacitance=1e-6  Setx0=off  InitialVoltage=0  Measurements=None
  Series RLC Branch10 : spsSeriesRLCBranchLib/Series RLC Branch  LConnTagsString=__new0  RConnTagsString=__new0  BranchType=RC  Resistance=0.0001  Inductance=20e-3  SetiL0=off  InitialCurrent=0  Capacitance=0.625e-6  Setx0=off  InitialVoltage=0  Measurements=None
  Series RLC Branch3 : spsSeriesRLCBranchLib/Series RLC Branch  LConnTagsString=__new0  RConnTagsString=__new0  BranchType=C  Resistance=1  Inductance=5e-3  SetiL0=off  InitialCurrent=0  Capacitance=30e-6  Setx0=off  InitialVoltage=0  Measurements=None
  Series RLC Branch4 : spsSeriesRLCBranchLib/Series RLC Branch  LConnTagsString=__new0  RConnTagsString=__new0  BranchType=C  Resistance=1  Inductance=5e-3  SetiL0=off  InitialCurrent=0  Capacitance=30e-6  Setx0=off  InitialVoltage=0  Measurements=None
  Series RLC Branch5 : spsSeriesRLCBranchLib/Series RLC Branch  LConnTagsString=__new0  RConnTagsString=__new0  BranchType=C  Resistance=1  Inductance=5e-3  SetiL0=off  InitialCurrent=0  Capacitance=30e-6  Setx0=off  InitialVoltage=0  Measurements=None
  Series RLC Branch9 : spsSeriesRLCBranchLib/Series RLC Branch  LConnTagsString=__new0  RConnTagsString=__new0  BranchType=RL  Resistance=0.0001  Inductance=20e-3  SetiL0=off  InitialCurrent=0  Capacitance=1e-6  Setx0=off  InitialVoltage=0  Measurements=None
  Subsystem : Subsystem
  Subsystem1 : Subsystem
      mask Display: image('Battery.jpg');
  Sum : Sum  Inputs=|-+
  Sum{1..2,5..6,8} (5 alike) : Sum  Inputs=|+-
  Sum3 : Sum  Inputs=|++
  Sum4 : Sum  Inputs=|++
  Sum7 : Sum  Inputs=|++
  Three-Phase Transformer (Two Windings) : spsThreePhaseTransformerTwoWindingsLib/Three-Phase Transformer (Two Windings)  Winding1Connection=Yg  Winding2Connection=Yg  CoreType=Three single-phase transformers  SetSaturation=off  Hysteresis=off  DataFile='hysteresis'  SetInitialFlux=off  Measurements=None  UNITS=pu  NominalPower=[ 25e6 , 50 ]  Winding1=[ 415 , 0.002 , 0.008 ]  Winding2=[ 25e3 , 0.002 , 0.008 ]  Rm=500  Lm=500  L0=0.5  Saturation=[ 0,0 ; 0.0024,1.2 ; 1.0,1.52 ]  InitialFluxes=[ 0.8 , -0.8 , 0.7 ]  BreakLoop=off  DiscreteSolver=Trapezoidal iterative  DataType=off  TransfoNumber=1
  Three-Phase V-I Measurement : spsThreePhaseVIMeasurementLib/Three-Phase V-I Measurement  VoltageMeasurement=phase-to-ground  SetLabelV=on  LabelV=VabcB  Vpu=off  VpuLL=off  CurrentMeasurement=no  SetLabelI=off  LabelI=Iabc  Ipu=on  Pbase=100e6  Vbase=500e3  OutputType=Complex  PhasorSimulation=off  PSBequivalent=0
  Three-Phase V-I Measurement1 : spsThreePhaseVIMeasurementLib/Three-Phase V-I Measurement  VoltageMeasurement=phase-to-ground  SetLabelV=off  LabelV=Vabc  Vpu=off  VpuLL=off  CurrentMeasurement=yes  SetLabelI=off  LabelI=Iabc  Ipu=off  Pbase=100e6  Vbase=500e3  OutputType=Complex  PhasorSimulation=off  PSBequivalent=0
  Three-Phase Breaker : spsThreePhaseBreakerLib/Three-Phase Breaker  InitialState=closed  SwitchA=on  SwitchB=on  SwitchC=on  SwitchTimes="[1/60  5/60]"  External=on  BreakerResistance=0.001  SnubberResistance=1e8  SnubberCapacitance=inf  Measurements=Breaker voltages and currents
  Unit Delay2 : UnitDelay  SampleTime=0.001  HasFrameUpgradeWarning=on
  Voltage Measurement : spsVoltageMeasurementLib/Voltage Measurement  PhasorSimulation=off  OutputType=Complex  PSBequivalent=0
  abc to Alpha-Beta-Zero : spsabctoAlphaBetaZeroLib/abc to Alpha-Beta-Zero
  abc to dq0 : spsabctodq0Lib/abc to dq0  Alignment=90 degrees behind phase A axis
  dq0 to abc : spsdq0toabcLib/dq0 to abc  Alignment=90 degrees behind phase A axis
  Connection Port : PMIOPort  Side=Right
  Connection Port1 : PMIOPort  Port=2  Side=Right
  Connection Port2 : PMIOPort  Port=3  Side=Right
  wires:
  [IQ] -> Gain/1
  Current Measurement1/1 -> [IY]
  PID Controller2/1 -> Sum3/1
  PWM Generator (DC-DC)/1 -> Logical Operator/1, [Buck]
  Sum1/1 -> PID Controller1/1
  Sum4/1 -> Gain1/1
  Gain1/1 -> Product/1
  [Boost] -> Mosfet1/1
  Sum/1 -> PID Controller/1
  Product/1 -> Mux1/1
  Demux3/1 -> [PWM1]
  [VD] -> Sum4/2
  abc to Alpha-Beta-Zero/1 -> [alphabeta], Alpha-Beta-Zero to dq0/1
  dq0 to abc/1 -> PWM Generator (2-Level)/1
  Demux1/1 -> [ID]
  Sum3/1 -> Sum4/1
  Product1/1 -> Mux1/2
  "Power (3ph, Instantaneous)"/2 -> Scope1/1
  [ID] -> Sum2/2
  [VDC] -> Scope4/1
  [VDC] -> Sum1/2
  Gain/1 -> Sum3/2
  [PWM4] -> Subsystem/4(PWM4)
  Mux1/1 -> dq0 to abc/1
  Current Measurement2/1 -> [IB]
  Demux/2 -> [VQ]
  Alpha-Beta-Zero to dq1/1 -> Demux2/1
  Alpha-Beta-Zero to dq0/1 -> Demux/1
  [PWM2] -> Subsystem/2(PWM2)
  [VabcB] -> "Power (3ph, Instantaneous)"/1, Scope2/1
  [IR] -> Mux2/1
  [IB] -> Mux/3
  Demux1/2 -> [IQ]
  Integrator/1 -> [wt], Alpha-Beta-Zero to dq1/2
  Demux3/3 -> [PWM3]
  Demux3/2 -> [PWM2]
  [IY] -> Mux/2
  [wt] -> abc to dq0/2
  Mux/1 -> abc to dq0/1
  [VDC] -> Product/2
  Constant3/1 -> Sum8/2
  Constant1/1 -> Sum1/1
  Sum7/1 -> Gain3/1
  [ID] -> Gain2/1
  Voltage Measurement/1 -> [VDC]
  "Power (3ph, Instantaneous)"/1 -> Scope/1
  Constant/1 -> Sum/2
  [wt] -> dq0 to abc/2
  Demux3/4 -> [PWM4]
  PID Controller4/1 -> PWM Generator (DC-DC)/1
  PID Controller/1 -> Integrator/1
  [alphabeta] -> Alpha-Beta-Zero to dq1/1
  Logical Operator/1 -> [Boost]
  Demux3/6 -> [PWM6]
  [IR] -> Mux/1
  Gain2/1 -> Sum6/2
  [VDC] -> Product1/2
  [Ibat] -> Sum8/1
  [VQ] -> Sum7/2
  Mux2/1 -> "Power (3ph, Instantaneous)"/2, Scope3/1
  Sum2/1 -> PID Controller2/1
  PID Controller3/1 -> Sum6/1
  [IQ] -> Sum5/2
  [IB] -> Mux2/3
  abc to dq0/1 -> Demux1/1
  [PWM5] -> Subsystem/5(PWM5)
  Current Measurement3/1 -> [IR]
  PID Controller1/1 -> Sum2/1
  Sum5/1 -> PID Controller3/1
  PWM Generator (2-Level)/1 -> Demux3/1
  [PWM6] -> Subsystem/6(PWM6)
  [PWM3] -> Subsystem/3(PWM3)
  [Ibat] -> Scope7/1
  Sum8/1 -> PID Controller4/1
  Gain3/1 -> Product1/1
  [IY] -> Mux2/2
  [Buck] -> Mosfet/1
  Demux2/2 -> Sum/1
  [PWM1] -> Subsystem/1(PWM1)
  [VabcB] -> abc to Alpha-Beta-Zero/1
  [SOC] -> Scope5/1
  Constant2/1 -> Sum5/1
  Demux3/5 -> [PWM5]
  Sum6/1 -> Sum7/1
  [wt] -> Alpha-Beta-Zero to dq0/2
  Demux/1 -> [VD]
  [Vbat] -> Scope6/1
  RMS/1 -> Display/1
  Three-Phase V-I Measurement1/1 -> Scope8/1
  Unit Delay2/1 -> Demux5/1
  Relay/1(Out1) -> Three-Phase Breaker/1
  Demux5/3 -> Relay/3(In3)
  Demux5/1 -> Relay/1(In1)
  Demux5/2 -> Relay/2(In2)
  Three-Phase V-I Measurement1/2 -> Scope8/2, RMS/1, Unit Delay2/1
  connections:
  Series RLC Branch5/LConn1 -- Series RLC Branch8/LConn1 -- Series RLC Branch2/RConn1
  Series RLC Branch9/RConn1 -- Series RLC Branch10/LConn1 -- Subsystem1/LConn1
  Series RLC Branch4/LConn1 -- Series RLC Branch7/LConn1 -- Series RLC Branch1/RConn1
  Series RLC Branch9/LConn1 -- Mosfet/RConn1 -- Mosfet1/LConn1
  Series RLC Branch3/LConn1 -- Series RLC Branch6/LConn1 -- Series RLC Branch/RConn1
  Mosfet1/RConn1 -- Subsystem/RConn2 -- Voltage Measurement/LConn2 -- Series RLC Branch10/RConn1 -- Subsystem1/LConn2
  Voltage Measurement/LConn1 -- Subsystem/RConn1 -- Mosfet/LConn1
  Series RLC Branch4/RConn1 -- Series RLC Branch5/RConn1 -- Series RLC Branch3/RConn1
  Series RLC Branch1/LConn1 -- Three-Phase V-I Measurement/RConn2
  Series RLC Branch8/RConn1 -- Current Measurement2/RConn1
  Subsystem/LConn1 -- Current Measurement3/LConn1
  Three-Phase V-I Measurement/LConn1 -- Three-Phase Transformer (Two Windings)/LConn1
  Subsystem/LConn3 -- Current Measurement2/LConn1
  Three-Phase V-I Measurement/LConn3 -- Three-Phase Transformer (Two Windings)/LConn3
  Three-Phase V-I Measurement/LConn2 -- Three-Phase Transformer (Two Windings)/LConn2
  Series RLC Branch6/RConn1 -- Current Measurement3/RConn1
  Series RLC Branch/LConn1 -- Three-Phase V-I Measurement/RConn1
  Current Measurement1/RConn1 -- Series RLC Branch7/RConn1
  Series RLC Branch2/LConn1 -- Three-Phase V-I Measurement/RConn3
  Subsystem/LConn2 -- Current Measurement1/LConn1
  Three-Phase V-I Measurement1/RConn1 -- Three-Phase Transformer (Two Windings)/RConn1
  Three-Phase V-I Measurement1/RConn2 -- Three-Phase Transformer (Two Windings)/RConn2
  Three-Phase V-I Measurement1/RConn3 -- Three-Phase Transformer (Two Windings)/RConn3
  Three-Phase Breaker/LConn1 -- Three-Phase V-I Measurement1/LConn1
  Three-Phase Breaker/LConn2 -- Three-Phase V-I Measurement1/LConn2
  Three-Phase Breaker/LConn3 -- Three-Phase V-I Measurement1/LConn3
  Connection Port/RConn1 -- Three-Phase Breaker/RConn1
  Connection Port1/RConn1 -- Three-Phase Breaker/RConn2
  Connection Port2/RConn1 -- Three-Phase Breaker/RConn3

== system Smart_Grid_2/Commercial Load ==
  Commercial Load : spsThreePhaseParallelRLCLoadLib/Three-Phase Parallel RLC Load  LConnTagsString=A|B|C  Configuration=Y (grounded)  NominalVoltage=25e3  Vabc=[1e3 1e3 1e3]  Vabcp=[1e3 1e3 1e3]  NominalFrequency=50  UnbalancedPower=off  ActivePower=50e3  InductivePower=100  CapacitivePower=7500  Pabc=[10e3 9e3 11e3]  QLabc=[100 90 110]  QCabc=[100 90 110]  Pabcp=[10e3 9e3 11e3]  QLabcp=[100 90 110]  QCabcp=[100 90 110]  Measurements=None  LoadType=constant Z
  Demux5 : Demux  Outputs=3
  "Power (3ph, Phasor)" : spsPower3phPhasorLib/Power (3ph, Phasor)
      settings: LibrarySourceBlock=|
      | sps_lib/Sensors and Measurements/Power
      | (3ph, Phasor)
  RMS : spsRMSLib/RMS  TrueRMS=on  Freq=60  RMSInit=120  Ts=0
  RMS1 : spsRMSLib/RMS  TrueRMS=on  Freq=60  RMSInit=120  Ts=0
  Relay : Subsystem
  Scope : Scope  NumInputPorts=2
  Three-Phase V-I Measurement6 : spsThreePhaseVIMeasurementLib/Three-Phase V-I Measurement  VoltageMeasurement=phase-to-ground  SetLabelV=off  LabelV=Commercial_Voltage  Vpu=off  VpuLL=off  CurrentMeasurement=yes  SetLabelI=off  LabelI=Commercial_Current  Ipu=off  Pbase=100e6  Vbase=500e3  OutputType=Complex  PhasorSimulation=off  PSBequivalent=0
  Three-Phase Breaker : spsThreePhaseBreakerLib/Three-Phase Breaker  InitialState=closed  SwitchA=on  SwitchB=on  SwitchC=on  SwitchTimes="[1/60  5/60]"  External=on  BreakerResistance=0.001  SnubberResistance=1e8  SnubberCapacitance=inf  Measurements=Breaker voltages and currents
  Unit Delay2 : UnitDelay  SampleTime=0.001  HasFrameUpgradeWarning=on
  A : PMIOPort  Side=Left
  B : PMIOPort  Port=2  Side=Left
  C : PMIOPort  Port=3  Side=Left
  wires:
  Unit Delay2/1 -> Demux5/1
  Relay/1(Out1) -> Three-Phase Breaker/1
  Demux5/3 -> Relay/3(In3)
  Demux5/1 -> Relay/1(In1)
  Demux5/2 -> Relay/2(In2)
  Three-Phase V-I Measurement6/2 -> "Power (3ph, Phasor)"/2, Unit Delay2/1
  Three-Phase V-I Measurement6/1 -> "Power (3ph, Phasor)"/1
  "Power (3ph, Phasor)"/1 -> RMS/1
  RMS/1 -> Scope/1
  "Power (3ph, Phasor)"/2 -> RMS1/1
  RMS1/1 -> Scope/2
  connections:
  Three-Phase V-I Measurement6/LConn1 -- A/RConn1
  Three-Phase V-I Measurement6/LConn2 -- B/RConn1
  Three-Phase V-I Measurement6/LConn3 -- C/RConn1
  Three-Phase Breaker/RConn1 -- Commercial Load/LConn1
  Three-Phase Breaker/RConn2 -- Commercial Load/LConn2
  Three-Phase Breaker/RConn3 -- Commercial Load/LConn3
  Three-Phase Breaker/LConn1 -- Three-Phase V-I Measurement6/RConn1
  Three-Phase Breaker/LConn2 -- Three-Phase V-I Measurement6/RConn2
  Three-Phase Breaker/LConn3 -- Three-Phase V-I Measurement6/RConn3

== system Smart_Grid_2/Industrial Load ==
  Demux5 : Demux  Outputs=3
  Industrial Load : spsThreePhaseParallelRLCLoadLib/Three-Phase Parallel RLC Load  LConnTagsString=A|B|C  Configuration=Y (grounded)  NominalVoltage=25e3  Vabc=[1e3 1e3 1e3]  Vabcp=[1e3 1e3 1e3]  NominalFrequency=50  UnbalancedPower=off  ActivePower=75e3  InductivePower=2500  CapacitivePower=6000  Pabc=[10e3 9e3 11e3]  QLabc=[100 90 110]  QCabc=[100 90 110]  Pabcp=[10e3 9e3 11e3]  QLabcp=[100 90 110]  QCabcp=[100 90 110]  Measurements=None  LoadType=constant Z
  "Power (3ph, Phasor)" : spsPower3phPhasorLib/Power (3ph, Phasor)
      settings: LibrarySourceBlock=|
      | sps_lib/Sensors and Measurements/Power
      | (3ph, Phasor)
  RMS : spsRMSLib/RMS  TrueRMS=on  Freq=60  RMSInit=120  Ts=0
  RMS1 : spsRMSLib/RMS  TrueRMS=on  Freq=60  RMSInit=120  Ts=0
  Relay : Subsystem
  Scope : Scope  NumInputPorts=2
  Three-Phase V-I Measurement8 : spsThreePhaseVIMeasurementLib/Three-Phase V-I Measurement  VoltageMeasurement=phase-to-ground  SetLabelV=off  LabelV=Industrial_Voltage  Vpu=off  VpuLL=off  CurrentMeasurement=yes  SetLabelI=off  LabelI=Industrial_Current  Ipu=off  Pbase=100e6  Vbase=500e3  OutputType=Complex  PhasorSimulation=off  PSBequivalent=0
  Three-Phase Breaker : spsThreePhaseBreakerLib/Three-Phase Breaker  InitialState=closed  SwitchA=on  SwitchB=on  SwitchC=on  SwitchTimes="[1/60  5/60]"  External=on  BreakerResistance=0.001  SnubberResistance=1e8  SnubberCapacitance=inf  Measurements=Breaker voltages and currents
  Unit Delay2 : UnitDelay  SampleTime=0.001  HasFrameUpgradeWarning=on
  C : PMIOPort  Side=Left
  B : PMIOPort  Port=2  Side=Left
  A : PMIOPort  Port=3  Side=Left
  wires:
  Demux5/1 -> Relay/1(In1)
  Unit Delay2/1 -> Demux5/1
  Three-Phase V-I Measurement8/1 -> "Power (3ph, Phasor)"/1
  Three-Phase V-I Measurement8/2 -> "Power (3ph, Phasor)"/2, Unit Delay2/1
  Demux5/2 -> Relay/2(In2)
  Relay/1(Out1) -> Three-Phase Breaker/1
  "Power (3ph, Phasor)"/2 -> RMS1/1
  Demux5/3 -> Relay/3(In3)
  RMS1/1 -> Scope/2
  "Power (3ph, Phasor)"/1 -> RMS/1
  RMS/1 -> Scope/1
  connections:
  Three-Phase V-I Measurement8/LConn1 -- A/RConn1
  Three-Phase V-I Measurement8/LConn2 -- B/RConn1
  Three-Phase V-I Measurement8/LConn3 -- C/RConn1
  Three-Phase Breaker/LConn2 -- Three-Phase V-I Measurement8/RConn2
  Three-Phase Breaker/RConn2 -- Industrial Load/LConn2
  Three-Phase Breaker/RConn1 -- Industrial Load/LConn1
  Three-Phase Breaker/LConn3 -- Three-Phase V-I Measurement8/RConn3
  Three-Phase Breaker/LConn1 -- Three-Phase V-I Measurement8/RConn1
  Three-Phase Breaker/RConn3 -- Industrial Load/LConn3

== system Smart_Grid_2/Residential Load 1 ==
  Demux5 : Demux  Outputs=3
  "Power (3ph, Phasor)" : spsPower3phPhasorLib/Power (3ph, Phasor)
      settings: LibrarySourceBlock=|
      | sps_lib/Sensors and Measurements/Power
      | (3ph, Phasor)
  RMS : spsRMSLib/RMS  TrueRMS=on  Freq=60  RMSInit=120  Ts=0
  RMS1 : spsRMSLib/RMS  TrueRMS=on  Freq=60  RMSInit=120  Ts=0
  Relay : Subsystem
  Residential Load 1 : spsThreePhaseParallelRLCLoadLib/Three-Phase Parallel RLC Load  LConnTagsString=A|B|C  Configuration=Y (grounded)  NominalVoltage=25e3  Vabc=[1e3 1e3 1e3]  Vabcp=[1e3 1e3 1e3]  NominalFrequency=50  UnbalancedPower=off  ActivePower=100e3  InductivePower=0  CapacitivePower=0  Pabc=[10e3 9e3 11e3]  QLabc=[100 90 110]  QCabc=[100 90 110]  Pabcp=[10e3 9e3 11e3]  QLabcp=[100 90 110]  QCabcp=[100 90 110]  Measurements=None  LoadType=constant Z
  Scope : Scope  NumInputPorts=2
  Three-Phase V-I Measurement7 : spsThreePhaseVIMeasurementLib/Three-Phase V-I Measurement  VoltageMeasurement=phase-to-ground  SetLabelV=off  LabelV=Residential_1_Voltage  Vpu=off  VpuLL=off  CurrentMeasurement=yes  SetLabelI=off  LabelI=Residential_1_Current  Ipu=off  Pbase=100e6  Vbase=500e3  OutputType=Complex  PhasorSimulation=off  PSBequivalent=0
  Three-Phase Breaker : spsThreePhaseBreakerLib/Three-Phase Breaker  InitialState=closed  SwitchA=on  SwitchB=on  SwitchC=on  SwitchTimes="[1/60  5/60]"  External=on  BreakerResistance=0.001  SnubberResistance=1e8  SnubberCapacitance=inf  Measurements=Breaker voltages and currents
  Unit Delay2 : UnitDelay  SampleTime=0.001  HasFrameUpgradeWarning=on
  A : PMIOPort  Side=Left
  B : PMIOPort  Port=2  Side=Left
  C : PMIOPort  Port=3  Side=Left
  wires:
  Three-Phase V-I Measurement7/2 -> "Power (3ph, Phasor)"/2, Unit Delay2/1
  RMS1/1 -> Scope/2
  RMS/1 -> Scope/1
  Demux5/1 -> Relay/1(In1)
  Demux5/2 -> Relay/2(In2)
  Demux5/3 -> Relay/3(In3)
  Relay/1(Out1) -> Three-Phase Breaker/1
  Unit Delay2/1 -> Demux5/1
  "Power (3ph, Phasor)"/2 -> RMS1/1
  Three-Phase V-I Measurement7/1 -> "Power (3ph, Phasor)"/1
  "Power (3ph, Phasor)"/1 -> RMS/1
  connections:
  Three-Phase V-I Measurement7/LConn1 -- A/RConn1
  Three-Phase V-I Measurement7/LConn3 -- C/RConn1
  Three-Phase V-I Measurement7/LConn2 -- B/RConn1
  Three-Phase Breaker/LConn1 -- Three-Phase V-I Measurement7/RConn1
  Three-Phase Breaker/LConn2 -- Three-Phase V-I Measurement7/RConn2
  Three-Phase Breaker/LConn3 -- Three-Phase V-I Measurement7/RConn3
  Three-Phase Breaker/RConn1 -- Residential Load 1/LConn1
  Three-Phase Breaker/RConn2 -- Residential Load 1/LConn2
  Three-Phase Breaker/RConn3 -- Residential Load 1/LConn3
